simulink model "Buck_Battery_PI-Control"  (R2019a)
settings: Solver=VariableStepAuto  StartTime=0.0  StopTime=2  RelTol=1e-3
undefined symbols (not defined in the file or in its folder): Acid, Down, Lead, Up
libraries: powerlib x9, powerlib_meascontrol x2, electricdrivelib x1, simulink x1, eePwmGenerator x1
settings Model: Creator=ryusl  LastModifiedBy=ryusl

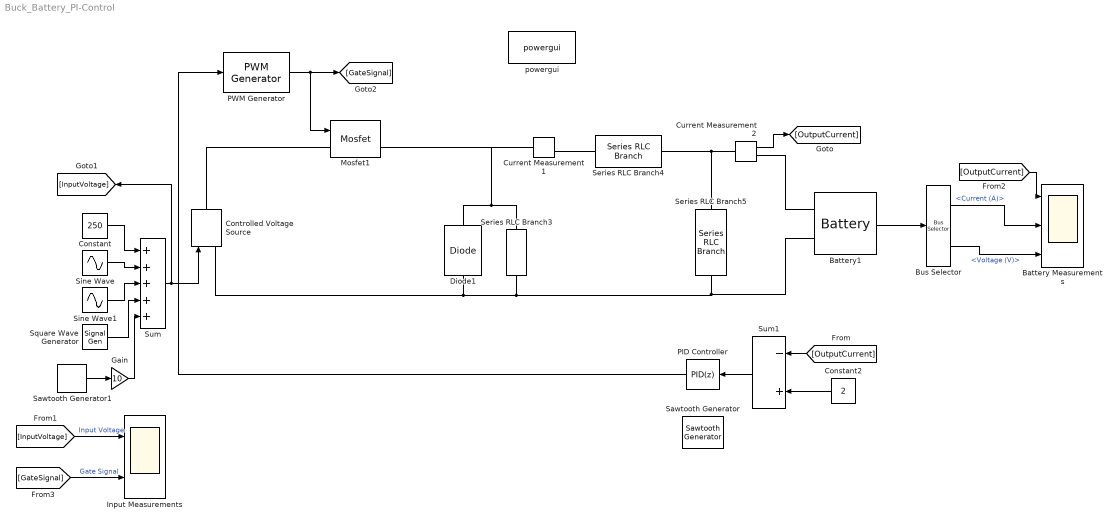
== system Buck_Battery_PI-Control ==
  Battery Measurements : Scope  NumInputPorts=3
  Battery1 : electricdrivelib/Extra Sources/Battery  BatType=Lead-Acid  ShowTempParam=off  ThermalPreset=no  ShowAgeParam=off  NomV=24  NomQ=13  SOC=50  Batt_Tr=0.000001  PresetModel=on  MaxQ=13.5417  MinV=18  FullV=26.1316  Dis_rate=2.6  R=0.018462  Normal_OP=4.0336  expZone="[24.4342    0.0433333]"  current=[6.5 13 32.5]  Units=Time  Tci=20  NomT=20  T2=-30  MaxQ2=4.8  FullV2=7.1  Normal_OP2=5.655  expZone2="[6.58           1]"  Rca=0.6  ti=2000  Dp=0  Neq0=0  Tsim=1e6  Ta1=25  Qeol=5.4*0.9  Reol=0.013333*1.2  Char_age=[2.3478, 3]  Dis_age=[2.3478, 10]  N1=1500  N2=10500  N3=1000  N4=1400  Ta2=45  N5=950
  Bus Selector : BusSelector  OutputSignals=Current (A),Voltage (V)
  Constant : Constant  Value=250
  Constant2 : Constant  Value=2
  Controlled Voltage Source : powerlib/Electrical Sources/Controlled Voltage Source  Initialize=on  Source_Type=AC  Amplitude=0  Phase=0  Frequency=0  Measurements=None
      settings: SourceProductName=Simscape Electrical
  Current Measurement1 : powerlib/Measurements/Current Measurement  PhasorSimulation=off  OutputType=Complex  PSBequivalent=0
  Current Measurement2 : powerlib/Measurements/Current Measurement  PhasorSimulation=off  OutputType=Complex  PSBequivalent=0
  Diode1 : powerlib/Power Electronics/Diode  Ron=0.001  Lon=0  Vf=0.001  IC=0  UseSnubber=0  Rs=0  Cs=0  Measurements=off
  Gain : Gain  Gain=10
  Input Measurements : Scope  NumInputPorts=2
  Mosfet1 : powerlib/Power Electronics/Mosfet  Ron=0.1  Lon=0  Rd=0.01  Vfd=1  IC=0  Rs=1e5  Cs=inf  Measurements=on
      settings: SourceProductName=Simscape Electrical
  PID Controller : simulink/Continuous/PID Controller  Controller=PID  Form=Parallel  TimeDomain=Discrete-time  SampleTime=5e-6  IntegratorMethod=Forward Euler  FilterMethod=Forward Euler  ControllerParametersSource=internal  P=100  I=200  D=0  UseFilter=off  N=100  TunerSelectOption=Transfer Function Based (PID Tuner App)  ZeroCross=off  InitialConditionSource=internal  InitialConditionForIntegrator=0  InitialConditionForFilter=0  DifferentiatorICPrevScaledInput=0  ExternalReset=none  TrackingMode=off  Kt=1  LimitOutput=off  UpperSaturationLimit=inf  LowerSaturationLimit=-inf  LinearizeAsGain=on  AntiWindupMode=none  Kb=1  POutMin=[]  POutMax=[]  IOutMin=[]  IOutMax=[]  DOutMin=[]  DOutMax=[]  NOutMin=[]  NOutMax=[]  SumOutMin=[]  SumOutMax=[]  SaturationOutMin=[]  SaturationOutMax=[]  PParamMin=[]  PParamMax=[]  IParamMin=[]  IParamMax=[]  DParamMin=[]  DParamMax=[]  NParamMin=[]  NParamMax=[]  KbParamMin=[]  KbParamMax=[]  KtParamMin=[]  KtParamMax=[]  KbOutMin=[]  KbOutMax=[]  KtOutMin=[]  KtOutMax=[]  IntegratorOutMin=[]  IntegratorOutMax=[]  FilterOutMin=[]  FilterOutMax=[]  SumI1OutMin=[]  SumI1OutMax=[]  SumI2OutMin=[]  SumI2OutMax=[]  SumI3OutMin=[]  SumI3OutMax=[]  SumI4OutMin=[]  SumI4OutMax=[]  SumDOutMin=[]  SumDOutMax=[]  DifferentiatorOutMin=[]  DifferentiatorOutMax=[]  FilterDiffOutCoefMin=[]  FilterDiffOutCoefMax=[]  ReciprocalOutMin=[]  ReciprocalOutMax=[]  SumDenOutMin=[]  SumDenOutMax=[]  SumNumOutMin=[]  SumNumOutMax=[]  DivideOutMin=[]  DivideOutMax=[]  IntegratorContinuousStateAttributes=''  IntegratorStateMustResolveToSignalObject=off  IntegratorRTWStateStorageClass=Auto  FilterContinuousStateAttributes=''  FilterStateMustResolveToSignalObject=off  FilterRTWStateStorageClass=Auto  ParallelPVariant=InternalParameters  IdealPVariant=Disabled  IVariant=InternalParameters  DVariant=InternalParameters  IntegratorVariant=Discrete  SatVariant=Disabled  AWVariant=Passthrough  PCopyVariant=Disabled  TRVariant=Disabled  FdbkBlocksVariant=Forward  IdealPFdbkVariant=Disabled  SatFdbkVariant=Disabled  DerivativeFilterVariant=Differentiator  NVariant=Passthrough  NCopyVariant=Disabled_SignalSpec  FilterICVariant=InternalICsDifferentiator  IntegratorICVariant=InternalICs  ExternalResetVariant=Disabled  TRSumVariant=Passthrough  SumFdbkVariant=Disabled  SumVariant=Sum_PID
  PWM Generator : eePwmGenerator/PWM Generator  CarrCount=Up-Down  Tper=1e-4  Ts=5e-6
  Sawtooth Generator : powerlib_meascontrol/Pulse & Signal Generators/Sawtooth Generator  Freq=1e4  Phase=180  Ts=5e-6
      settings: SourceProductName=Simscape Electrical
  Sawtooth Generator1 : powerlib_meascontrol/Pulse & Signal Generators/Sawtooth Generator  Freq=100  Phase=180  Ts=1e-5
      settings: SourceProductName=Simscape Electrical
  Series RLC Branch3 : powerlib/Elements/Series RLC Branch  LConnTagsString=__new0  RConnTagsString=__new0  BranchType=R  Resistance=1e6  Inductance=1e-3  SetiL0=off  InitialCurrent=0  Capacitance=1e-6  Setx0=off  InitialVoltage=0  Measurements=None
  Series RLC Branch4 : powerlib/Elements/Series RLC Branch  LConnTagsString=__new0  RConnTagsString=__new0  BranchType=L  Resistance=1  Inductance=0.01223  SetiL0=off  InitialCurrent=0  Capacitance=1e-6  Setx0=off  InitialVoltage=0  Measurements=None
  Series RLC Branch5 : powerlib/Elements/Series RLC Branch  LConnTagsString=__new0  RConnTagsString=__new0  BranchType=RC  Resistance=0.2  Inductance=1e-9  SetiL0=off  InitialCurrent=0  Capacitance=1.63e-6  Setx0=on  InitialVoltage=24.1  Measurements=None
  Sine Wave : Sin  Amplitude=50  Frequency=10  SampleTime=1e-5
  Sine Wave1 : Sin  Amplitude=30  Frequency=10  Phase=1  SampleTime=1e-5
  Square Wave Generator : SignalGenerator  WaveForm=random  Amplitude=10  Frequency=15  Units=rad/sec
  Sum : Sum  Inputs=+++++
  Sum1 : Sum  Inputs=-+
  powergui : powerlib/powergui  Priority=1  SimulationMode=Discrete  SampleTime=5e-6  frequency=60  Iterations=50  frequencyindice=0  Pbase=100e6  ErrMax=1e-4  UnitsV=kV  UnitsW=MW  buscounter=0  FunctionMessages=off  echomessages=off  EnableUseOfTLC=off  CurrentSourceSwitches=off  DisableSnubberDevices=off  DisableRonSwitches=off  DisableVfSwitches=off  DisplayEquations=off  AutomaticDiscreteSolvers=off  SolverType=Tustin/Backward Euler (TBE)  Interpol=off  ExternalGateDelay=off  methode=off  Ts=100  x0status=blocks  SPID=on  SwTol=0  HookPort=off  NonlinearTolerance=1e-4  nMaxIteration=100  ContinueOnMaxIteration=off  RestoreLinks=warning  ResistiveCurrentMeasurement=off  Frange=[0:2:500]  Ylog=off  Xlog=on  ShowGrid=off  save=off  variable=ZData  structure=0  ZoomFFT=off  StartTime=0.0  cycles=1  DisplayStyle=1  fundamental=60  FreqAxis=off  MaxFrequency=1000  frequencyindicesteady=1  RmsSteady=1  display=off
  wires:
  Battery1/1 -> Bus Selector/1
  PWM Generator/1 -> Mosfet1/1, [GateSignal]
  Current Measurement2/1 -> [OutputCurrent]
  [OutputCurrent] -> Sum1/1
  Constant2/1 -> Sum1/2
  Sum1/1 -> PID Controller/1
  PID Controller/1 -> PWM Generator/1
  Bus Selector/1 -> Battery Measurements/2  "<Current (A)>"
  Bus Selector/2 -> Battery Measurements/3  "<Voltage (V)>"
  [InputVoltage] -> Input Measurements/1  "Input Voltage"
  [OutputCurrent] -> Battery Measurements/1
  Sine Wave/1 -> Sum/2
  Sine Wave1/1 -> Sum/3
  Constant/1 -> Sum/1
  Square Wave Generator/1 -> Sum/4
  Sum/1 -> [InputVoltage], Controlled Voltage Source/1
  Sawtooth Generator1/1 -> Gain/1
  Gain/1 -> Sum/5
  [GateSignal] -> Input Measurements/2  "Gate Signal"
  connections:
  Diode1/RConn1 -- Current Measurement1/LConn1 -- Mosfet1/RConn1 -- Series RLC Branch3/LConn1
  Diode1/LConn1 -- Battery1/LConn2 -- Series RLC Branch5/RConn1 -- Series RLC Branch3/RConn1 -- Controlled Voltage Source/LConn1
  Series RLC Branch4/RConn1 -- Current Measurement2/LConn1 -- Series RLC Branch5/LConn1
  Current Measurement1/RConn1 -- Series RLC Branch4/LConn1
  Controlled Voltage Source/RConn1 -- Mosfet1/LConn1
  Current Measurement2/RConn1 -- Battery1/LConn1
